simulink model "Evaporator_dummy_linearized_0"  (R2025b)
settings: Solver=VariableStepAuto  StartTime=0.0  StopTime=10.0  RelTol=1e-3
settings Model: Creator=malcolmrenney  LastModifiedBy=malcolmrenney

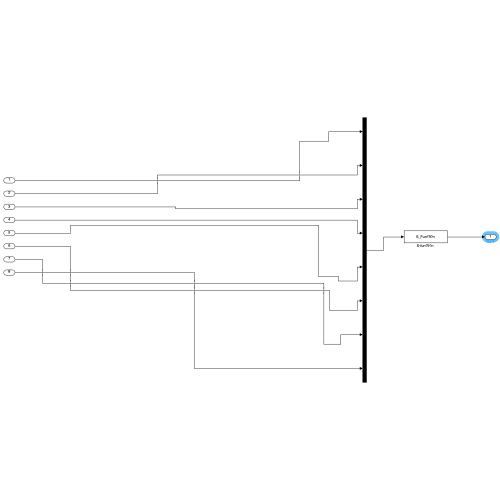
[thumbnail: Simulink's stored preview of the top-level diagram]
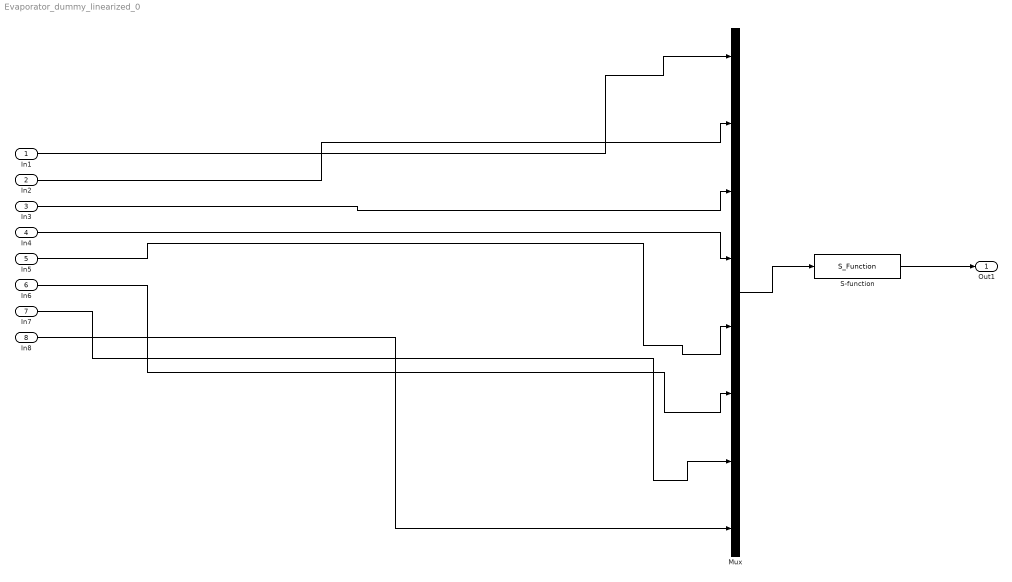
== system Evaporator_dummy_linearized_0 ==
  In1 : Inport
  In2 : Inport  Port=2
  In3 : Inport  Port=3
  In4 : Inport  Port=4
  In5 : Inport  Port=5
  In6 : Inport  Port=6
  In7 : Inport  Port=7
  In8 : Inport  Port=8
  Mux : Mux  Inputs=8
  "S-function " : S-Function  FunctionName=S_Function  Parameters=xinit, par  SFunctionDeploymentMode=off  EnableBusSupport=off
  Out1 : Outport
  wires:
  In7/1 -> Mux/7
  In6/1 -> Mux/6
  In4/1 -> Mux/4
  In2/1 -> Mux/2
  In3/1 -> Mux/3
  In1/1 -> Mux/1
  In5/1 -> Mux/5
  In8/1 -> Mux/8
  Mux/1 -> "S-function "/1
  "S-function "/1 -> Out1/1
